simulink model "MySimModel"  (R2024b)
settings: Solver=VariableStepAuto  StartTime=0.0  StopTime=10.0  RelTol=1e-3
settings Model: Creator=xinxing  LastModifiedBy=xinxing

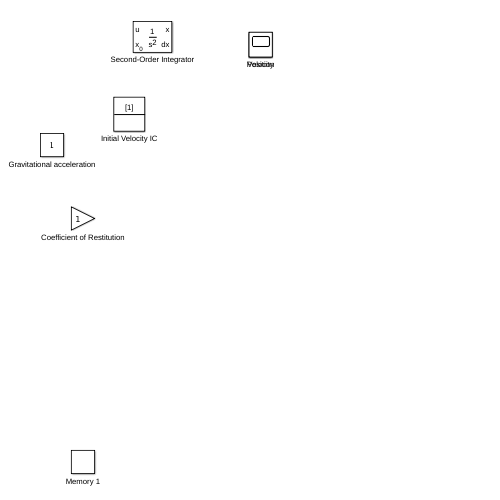
[thumbnail: Simulink's stored preview of the top-level diagram]
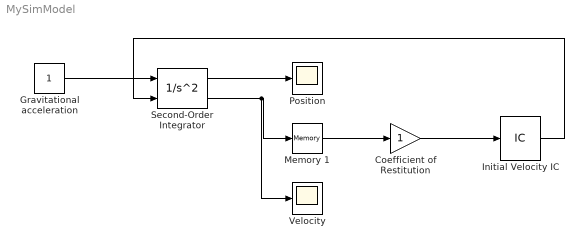
== system MySimModel ==
  Coefficient of Restitution : Gain
  Gravitational acceleration : Constant
  Initial Velocity IC : InitialCondition
  Memory 1 : Memory
  Position : Scope
  Second-Order Integrator : SecondOrderIntegrator  ICSourceX=external
  Velocity : Scope
  wires:
  Initial Velocity IC/1 -> Second-Order Integrator/2
  Memory 1/1 -> Coefficient of Restitution/1
  Coefficient of Restitution/1 -> Initial Velocity IC/1
  Second-Order Integrator/2 -> Memory 1/1, Velocity/1
  Second-Order Integrator/1 -> Position/1
  Gravitational acceleration/1 -> Second-Order Integrator/1
